simulink model "Microgrid_Islanding"  (R2025a)
settings: Solver=VariableStepAuto  StartTime=0.0  StopTime=5  RelTol=1e-3
settings Model: Creator=ASUS  LastModifiedBy=ASUS

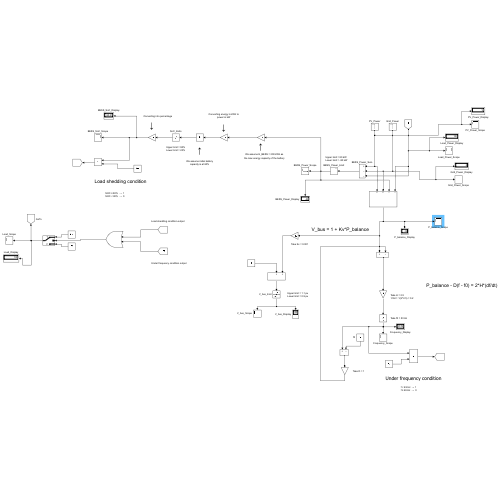
[thumbnail: Simulink's stored preview of the top-level diagram]
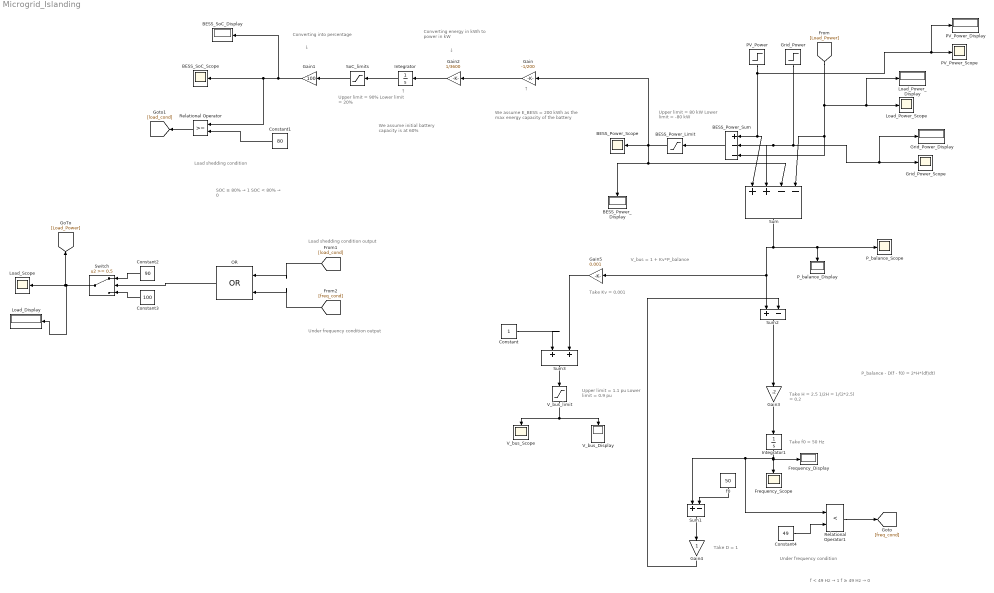
== system Microgrid_Islanding ==
  note: Under frequency condition output
  note: Load shedding condition output
  note: f < 49 Hz  → 1
      | f ≥ 49 Hz  →  0
  note: SOC ≥ 80%  →  1
      | SOC < 80%  →  0
  note: Under frequency condition
  note: Load shedding condition
  note: Upper limit = 90%
      | Lower limit = 20%
  note: Upper limit = 1.1 pu
      | Lower limit = 0.9 pu
  note: Upper limit = 80 kW
      | Lower limit = -80 kW
  note: Take Kv = 0.001
  note: V_bus = 1 + Kv*P_balance
  note: Take D = 1
  note: Take f0 = 50 Hz
  note: Take H = 2.5
      | 1/2H = 1/(2*2.5) = 0.2
  note: P_balance - D(f - f0) = 2*H*(df/dt)
  note: ↓
  note: We assume E_BESS = 200 kWh as
      | the max energy capacity of the battery
  note: ↓
  note: We assume initial battery
      | capacity is at 60%
  note: ↑
  note: ↑
  note: Converting into percentage
  note: Converting energy in kWh to
      | power in kW
  BESS_Power_Display : Display
  BESS_Power_Limit : Saturate  UpperLimit=80  LowerLimit=-80
  BESS_Power_Scope : Scope
      settings: ActiveDisplayYMinimum=-147.973265646472  ActiveDisplayYMaximum=368.275805795094  DataLoggingVariableName=ScopeData2
  BESS_Power_Sum : Sum  Inputs=+--
  BESS_SoC_Display : Display
  BESS_SoC_Scope : Scope
      settings: ActiveDisplayYMinimum=59.98770930530263  ActiveDisplayYMaximum=60.027998782142667
  Constant : Constant
  Constant1 : Constant  Value=80
  Constant2 : Constant  Value=90
  Constant3 : Constant  Value=100
  Constant4 : Constant  Value=49
  Frequency_Display : Display
  Frequency_Scope : Scope
      settings: ActiveDisplayYMinimum=41.565274060975007  ActiveDisplayYMaximum=90.10235160353713  DataLoggingVariableName=ScopeData3
  Gain : Gain  Gain=-1/200
  Gain1 : Gain  Gain=100
  Gain2 : Gain  Gain=1/3600
  Gain3 : Gain  Gain=.2
  Gain4 : Gain
  Gain5 : Gain  Gain=0.001
  Grid_Power : Step  Time=2  Before=50  After=0  SampleTime=0
  Grid_Power_Display : Display
  Grid_Power_Scope : Scope
      settings: ActiveDisplayYMinimum=-7.93340023657284  ActiveDisplayYMaximum=58.070617739613034  DataLoggingVariableName=ScopeData7
  Integrator : Integrator  InitialCondition=.6
  Integrator1 : Integrator  InitialCondition=50
  Load_Display : Display
  Load_Power_Display : Display
  Load_Power_Scope : Scope
      settings: ActiveDisplayYMinimum=-1  ActiveDisplayYMaximum=1  DataLoggingVariableName=ScopeData6
  Load_Scope : Scope
      settings: ActiveDisplayYMinimum=87.754147958276917  ActiveDisplayYMaximum=102.47663167587821  DataLoggingVariableName=ScopeData5
  OR : Logic  Operator=OR  IconShape=distinctive  AllPortsSameDT=off  OutDataTypeStr=boolean
  PV_Power : Step  Time=2  Before=100  After=10  SampleTime=0
  PV_Power_Display : Display
  PV_Power_Scope : Scope
      settings: ActiveDisplayYMinimum=-1  ActiveDisplayYMaximum=1  DataLoggingVariableName=ScopeData8
  P_balance_Display : Display
  P_balance_Scope : Scope
      settings: ActiveDisplayYMinimum=-106.20134067183822  ActiveDisplayYMaximum=272.29267080262571
  Relational Operator : RelationalOperator  OutDataTypeStr=boolean  RndMeth=Simplest  InputSameDT=off
  Relational Operator1 : RelationalOperator  Operator=<  OutDataTypeStr=boolean  ZeroCross=off  RndMeth=Simplest  InputSameDT=off
  SoC_limits : Saturate  UpperLimit=0.9  LowerLimit=0.2
  Sum : Sum  Inputs=|++--
  Sum1 : Sum  Inputs=+-
  Sum2 : Sum  Inputs=+-
  Sum3 : Sum  Inputs=|++
  Switch : Switch  Threshold=0.5  SaturateOnIntegerOverflow=off  InputSameDT=off
  V_bus_Display : Display
  V_bus_Scope : Scope
      settings: ActiveDisplayYMinimum=-1  ActiveDisplayYMaximum=1  DataLoggingVariableName=ScopeData4
  V_bus_limit : Saturate  UpperLimit=1.1  LowerLimit=0.9
  f0 : Constant  Value=50
  wires:
  PV_Power/1 -> PV_Power_Display/1, PV_Power_Scope/1, Sum/1, BESS_Power_Sum/1
  [Load_Power] -> Load_Power_Scope/1, Load_Power_Display/1, Sum/4, BESS_Power_Sum/3
  Sum/1 -> Gain5/1, Sum2/1, P_balance_Scope/1, P_balance_Display/1
  Grid_Power/1 -> Grid_Power_Display/1, Grid_Power_Scope/1, BESS_Power_Sum/2, Sum/2
  BESS_Power_Sum/1 -> BESS_Power_Limit/1
  Gain2/1 -> Integrator/1
  Gain/1 -> Gain2/1
  Gain1/1 -> BESS_SoC_Display/1, Relational Operator/1, BESS_SoC_Scope/1
  Integrator/1 -> SoC_limits/1
  Gain3/1 -> Integrator1/1
  Integrator1/1 -> Relational Operator1/1, Sum1/1, Frequency_Scope/1, Frequency_Display/1
  f0/1 -> Sum1/2
  Sum1/1 -> Gain4/1
  Sum2/1 -> Gain3/1
  Gain4/1 -> Sum2/2
  BESS_Power_Limit/1 -> Gain/1, BESS_Power_Scope/1, Sum/3, BESS_Power_Display/1
  Gain5/1 -> Sum3/2
  Constant/1 -> Sum3/1
  Sum3/1 -> V_bus_limit/1
  V_bus_limit/1 -> V_bus_Display/1, V_bus_Scope/1
  SoC_limits/1 -> Gain1/1
  Constant3/1 -> Switch/3
  Constant2/1 -> Switch/1
  Constant1/1 -> Relational Operator/2
  Switch/1 -> [Load_Power], Load_Scope/1, Load_Display/1
  Constant4/1 -> Relational Operator1/2
  Relational Operator1/1 -> [freq_cond]
  Relational Operator/1 -> [load_cond]
  OR/1 -> Switch/2
  [load_cond] -> OR/1
  [freq_cond] -> OR/2
